simulink model "Ship_Control_Loop_H_Infinity_Standard_Controller_Comparison"  (R2024a)
settings: Solver=VariableStepAuto  StartTime=0.0  StopTime=150  RelTol=1e-3
values from neighbouring files (symbols this model uses):
  Controller = Corrector_After_Reduction    [Aposteriori_Corrector_Order_Reduction.m]    (also in Standard_H_Infinity_Controller_Tuning.m = minreal(Controller))
  Input_Matrix_Controller_Nominal = Input_Matrix_Controller_After_Reduction    [Aposteriori_Corrector_Order_Reduction.m]
  Input_Measurement_Matrix_Controller_Nominal = Input_Measurement_Matrix_Controller_After_Reduction    [Aposteriori_Corrector_Order_Reduction.m]
  Measurement_Matrix_Controller_Nominal = Measurement_Matrix_Controller_After_Reduction    [Aposteriori_Corrector_Order_Reduction.m]
  Perturbation_Step = 10*(pi/180)    (= 0.174532925199)    [Controller_Stochastic_Optimization.m]    (also in Frequency_Responses.m)
  State_Matrix_Controller_Nominal = State_Matrix_Controller_After_Reduction    [Aposteriori_Corrector_Order_Reduction.m]
  Step_Heading_Aimed = 30*(pi/180)    (= 0.523598775598)    [Controller_Stochastic_Optimization.m]    (also in Frequency_Responses.m)
libraries: cstblocks x2, RCTblocks x2
settings Model: Creator=gerar  LastModifiedBy=gerar

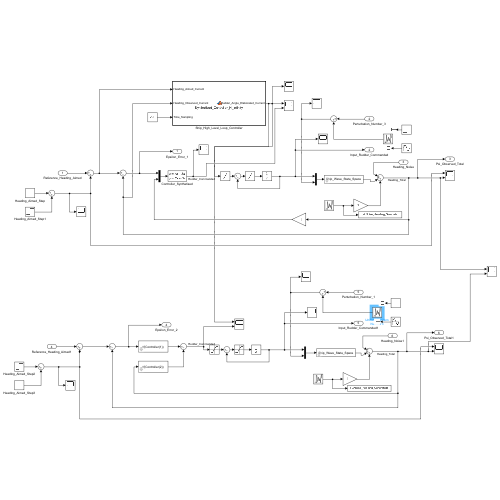
[thumbnail: Simulink's stored preview of the top-level diagram]
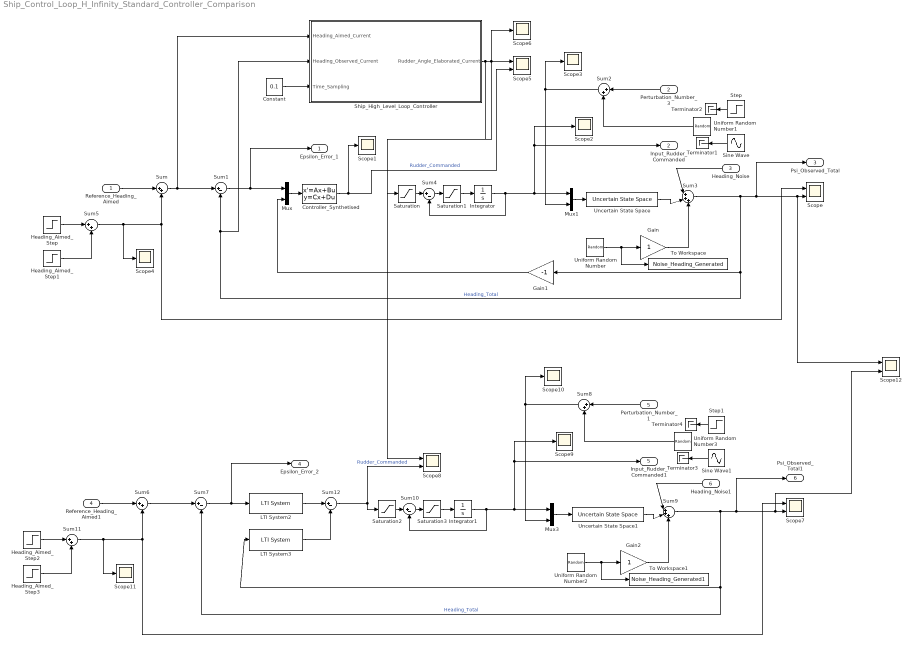
== system Ship_Control_Loop_H_Infinity_Standard_Controller_Comparison ==
  Reference_Heading_Aimed : Inport
  Perturbation_Number_3 : Inport  Port=2
  Heading_Noise : Inport  Port=3
  Reference_Heading_Aimed1 : Inport  Port=4
  Perturbation_Number_1 : Inport  Port=5
  Heading_Noise1 : Inport  Port=6
  Constant : Constant  Value=0.1
  Controller_Synthetised : StateSpace  A=State_Matrix_Controller_Nominal  B=Input_Matrix_Controller_Nominal  C=Measurement_Matrix_Controller_Nominal  D=Input_Measurement_Matrix_Controller_Nominal  InitialCondition=0
  Gain : Gain  SaturateOnIntegerOverflow=on  OutDataTypeStr=Inherit: Same as input  ParamDataTypeStr=Inherit: Same as input
  Gain1 : Gain  Gain=-1  SaturateOnIntegerOverflow=on  OutDataTypeStr=Inherit: Same as input  ParamDataTypeStr=Inherit: Same as input
  Gain2 : Gain  SaturateOnIntegerOverflow=on  OutDataTypeStr=Inherit: Same as input  ParamDataTypeStr=Inherit: Same as input
  Heading_Aimed_Step : Step  Time=0  After=Step_Heading_Aimed  SampleTime=0
  Heading_Aimed_Step1 : Step  Time=20  After=50*(pi/180)  SampleTime=0
  Heading_Aimed_Step2 : Step  Time=0  After=Step_Heading_Aimed  SampleTime=0
  Heading_Aimed_Step3 : Step  Time=20  After=50*(pi/180)  SampleTime=0
  Integrator : Integrator
  Integrator1 : Integrator
  LTI System2 : cstblocks/LTI System  sys=tf(Controller(1))  IC=[]  PadeOrder=0
  LTI System3 : cstblocks/LTI System  sys=tf(Controller(2))  IC=[]  PadeOrder=0
  Mux : Mux  Inputs=2
  Mux1 : Mux  Inputs=2
  Mux3 : Mux  Inputs=2
  Saturation : Saturate  UpperLimit=35*(pi/180)  LowerLimit=-35*(pi/180)
  Saturation1 : Saturate  UpperLimit=8*(pi/180)  LowerLimit=-8*(pi/180)
  Saturation2 : Saturate  UpperLimit=35*(pi/180)  LowerLimit=-35*(pi/180)
  Saturation3 : Saturate  UpperLimit=8*(pi/180)  LowerLimit=-8*(pi/180)
  Scope{,5,7..8,12} (5 alike) : Scope  NumInputPorts=2
  Scope{1..4,6,9..11} (8 alike) : Scope
  Ship_High_Level_Loop_Controller : MATLAB Function  TreatAsAtomicUnit=on  SystemSampleTime=0.1
  Sine Wave : Sin  Amplitude=2*(pi/180)  Frequency=0.6  SampleTime=0
  Sine Wave1 : Sin  Amplitude=2*(pi/180)  Frequency=0.6  SampleTime=0
  Step : Step  Time=10  After=Perturbation_Step  SampleTime=0
  Step1 : Step  Time=10  After=Perturbation_Step  SampleTime=0
  Sum{,2,5..6,8,11} (6 alike) : Sum  Inputs=|++
  Sum{1,4,7,10,12} (5 alike) : Sum  Inputs=|+-
  Sum3 : Sum  Inputs=|+++
  Sum9 : Sum  Inputs=|+++
  Terminator{1..4} (4 alike) : Terminator
  To Workspace : ToWorkspace  VariableName=Noise_Heading_Generated  SaveFormat=Timeseries  SampleTime=-1
  To Workspace1 : ToWorkspace  VariableName=Noise_Heading_Generated1  SaveFormat=Timeseries  SampleTime=-1
  Uncertain State Space : RCTblocks/Uncertain State Space  Tag=USS  USystem=Ship_Wave_State_Space  UValue=[]  X0=[]  uX0=[]
  Uncertain State Space1 : RCTblocks/Uncertain State Space  Tag=USS  USystem=Ship_Wave_State_Space  UValue=[]  X0=[]  uX0=[]
  Uniform Random Number : UniformRandomNumber  Minimum=-0.5*(pi/180)  Maximum=0.5*(pi/180)  SampleTime=1e-2
  Uniform Random Number1 : UniformRandomNumber  Minimum=-15*(pi/180)  Maximum=15*(pi/180)  SampleTime=1e-2
  Uniform Random Number2 : UniformRandomNumber  Minimum=-0.5*(pi/180)  Maximum=0.5*(pi/180)  SampleTime=1e-2
  Uniform Random Number3 : UniformRandomNumber  Minimum=-15*(pi/180)  Maximum=15*(pi/180)  SampleTime=1e-2
  Epsilon_Error_1 : Outport
  Input_Rudder_Commanded : Outport  Port=2
  Psi_Observed_Total : Outport  Port=3
  Epsilon_Error_2 : Outport  Port=4
  Input_Rudder_Commanded1 : Outport  Port=5
  Psi_Observed_Total1 : Outport  Port=6
  wires:
  Reference_Heading_Aimed/1 -> Sum/1
  Sum/1 -> Ship_High_Level_Loop_Controller/1(Heading_Aimed_Current), Sum1/1
  Sum1/1 -> Epsilon_Error_1/1, Mux/1
  Mux/1 -> Controller_Synthetised/1
  Controller_Synthetised/1 -> Scope5/2, Scope1/1  "Rudder_Commanded"
  Perturbation_Number_3/1 -> Sum2/1
  Sum2/1 -> Scope3/1, Mux1/2
  Mux1/1 -> Uncertain State Space/1
  Uncertain State Space/1 -> Sum3/2
  Heading_Noise/1 -> Sum3/1
  Uniform Random Number/1 -> To Workspace/1, Gain/1
  Gain/1 -> Sum3/3
  Sum3/1 -> Gain1/1, Ship_High_Level_Loop_Controller/2(Heading_Observed_Current), Sum1/2, Psi_Observed_Total/1, Scope12/1, Scope/2  "Heading_Total"
  Gain1/1 -> Mux/2
  Saturation1/1 -> Integrator/1
  Integrator/1 -> Sum4/2, Scope2/1, Input_Rudder_Commanded/1, Mux1/1
  Saturation/1 -> Sum4/1
  Sum4/1 -> Saturation1/1
  Sine Wave/1 -> Terminator1/1
  Uniform Random Number1/1 -> Sum2/2
  Step/1 -> Terminator2/1
  Heading_Aimed_Step/1 -> Sum5/1
  Heading_Aimed_Step1/1 -> Sum5/2
  Sum5/1 -> Scope4/1, Sum/2, Scope/1
  Constant/1 -> Ship_High_Level_Loop_Controller/3(Time_Sampling)
  Ship_High_Level_Loop_Controller/1(Rudder_Angle_Elaborated_Current) -> Scope8/1, Saturation/1, Scope5/1, Scope6/1
  Mux3/1 -> Uncertain State Space1/1
  Sum11/1 -> Scope11/1, Sum6/2, Scope7/1
  Uniform Random Number2/1 -> To Workspace1/1, Gain2/1
  Heading_Noise1/1 -> Sum9/1
  Uncertain State Space1/1 -> Sum9/2
  Gain2/1 -> Sum9/3
  Heading_Aimed_Step3/1 -> Sum11/2
  Saturation2/1 -> Sum10/1
  Saturation3/1 -> Integrator1/1
  Step1/1 -> Terminator4/1
  Uniform Random Number3/1 -> Sum8/2
  Sum12/1 -> Saturation2/1, Scope8/2  "Rudder_Commanded"
  Reference_Heading_Aimed1/1 -> Sum6/1
  Perturbation_Number_1/1 -> Sum8/1
  Sum7/1 -> Epsilon_Error_2/1, LTI System2/1
  Sum8/1 -> Scope10/1, Mux3/2
  Sum6/1 -> Sum7/1
  Integrator1/1 -> Sum10/2, Scope9/1, Input_Rudder_Commanded1/1, Mux3/1
  Sum10/1 -> Saturation3/1
  Sum9/1 -> LTI System3/1, Sum7/2, Psi_Observed_Total1/1, Scope12/2, Scope7/2  "Heading_Total"
  Sine Wave1/1 -> Terminator3/1
  Heading_Aimed_Step2/1 -> Sum11/1
  LTI System3/1 -> Sum12/2
  LTI System2/1 -> Sum12/1

== matlab function Ship_Control_Loop_H_Infinity_Standard_Controller_Comparison/Ship_High_Level_Loop_Controller ==
  data: Heading_Aimed_Current input; Rudder_Angle_Elaborated_Current output; Heading_Observed_Current input; Time_Sampling input
function Rudder_Angle_Elaborated_Current = Synthetized_Controller_H_Infinity(Heading_Aimed_Current,...
                                                                             Heading_Observed_Current,...
                                                                             Time_Sampling)


% This controller is based on the stochastic optimization done to find
% optimal parameters for the reduced controller of order 3 with two degrees
% of freedom.
% Heading observed persistents:
persistent Heading_Observed_Previous;
persistent Heading_Observed_Previous_Previous;
persistent Heading_Observed_Previous_Previous_Previous;
% Heading aimed persistents:
persistent Heading_Aimed_Previous;
persistent Heading_Aimed_Previous_Previous;
persistent Heading_Aimed_Previous_Previous_Previous;
% Rudder persistents:
persistent Rudder_Transfer_1_Previous;
persistent Rudder_Transfer_1_Previous_Previous;
persistent Rudder_Transfer_1_Previous_Previous_Previous;
persistent Rudder_Transfer_2_Previous;
persistent Rudder_Transfer_2_Previous_Previous;
persistent Rudder_Transfer_2_Previous_Previous_Previous;

% Persistents initialization:
if isempty(Heading_Observed_Previous)
    Heading_Observed_Previous = 0;
    Heading_Observed_Previous_Previous = 0;
    Heading_Observed_Previous_Previous_Previous = 0;
end
if isempty(Heading_Aimed_Previous)
    Heading_Aimed_Previous = 0;
    Heading_Aimed_Previous_Previous = 0;
    Heading_Aimed_Previous_Previous_Previous = 0;
end
if isempty(Rudder_Transfer_1_Previous)
    Rudder_Transfer_1_Previous = 0;
    Rudder_Transfer_1_Previous_Previous = 0;
    Rudder_Transfer_1_Previous_Previous_Previous = 0;
end
if isempty(Rudder_Transfer_2_Previous)
    Rudder_Transfer_2_Previous = 0;
    Rudder_Transfer_2_Previous_Previous = 0;
    Rudder_Transfer_2_Previous_Previous_Previous = 0;
end

% Tustin sampling:
Tustin_Sampling = 2/Time_Sampling;

% Controller coefficients:
% Numerator_Coefficient_Controller_1_1 = -1.663e-05;
% Numerator_Coefficient_Controller_1_2 = -0.4395;
% Numerator_Coefficient_Controller_1_3 = -3.978;
% Numerator_Coefficient_Controller_1_4 = -0.178;
% Denominator_Coefficient_Controller_1_1 = 1;
% Denominator_Coefficient_Controller_1_2 = 12.05;
% Denominator_Coefficient_Controller_1_3 = 14.03;
% Denominator_Coefficient_Controller_1_4 = 8.131;
% 
% Numerator_Coefficient_Controller_2_1 = -0.00014;
% Numerator_Coefficient_Controller_2_2 = -1.349;
% Numerator_Coefficient_Controller_2_3 = -17.03;
% Numerator_Coefficient_Controller_2_4 = 0.0001091;
% Denominator_Coefficient_Controller_2_1 = 1;
% Denominator_Coefficient_Controller_2_2 = 12.05;
% Denominator_Coefficient_Controller_2_3 = 14.03;
% Denominator_Coefficient_Controller_2_4 = 8.131;

Numerator_Coefficient_Controller_1_1 = 4.251e-05;
Numerator_Coefficient_Controller_1_2 = -1.03;
Numerator_Coefficient_Controller_1_3 = -1.866;
Numerator_Coefficient_Controller_1_4 = -0.1164;
Denominator_Coefficient_Controller_1_1 = 1;
Denominator_Coefficient_Controller_1_2 = 3.259;
Denominator_Coefficient_Controller_1_3 = 3.782;
Denominator_Coefficient_Controller_1_4 = 1.992;

Numerator_Coefficient_Controller_2_1 = 6.017e-05;
Numerator_Coefficient_Controller_2_2 = -2.254;
Numerator_Coefficient_Controller_2_3 = -3.937;
Numerator_Coefficient_Controller_2_4 = -6.421e-05;
Denominator_Coefficient_Controller_2_1 = 1;
Denominator_Coefficient_Controller_2_2 = 3.259;
Denominator_Coefficient_Controller_2_3 = 3.782;
Denominator_Coefficient_Controller_2_4 = 1.992;


% Coefficients calculation:
% First degree of freedom corrector:
Alpha_01 = Numerator_Coefficient_Controller_1_1*Tustin_Sampling^3 + Numerator_Coefficient_Controller_1_2*Tustin_Sampling^2 +...
           Numerator_Coefficient_Controller_1_3*Tustin_Sampling + Numerator_Coefficient_Controller_1_4;
Alpha_11 = -3*Numerator_Coefficient_Controller_1_1*Tustin_Sampling^3 - Numerator_Coefficient_Controller_1_2*Tustin_Sampling^2 +...
           Numerator_Coefficient_Controller_1_3*Tustin_Sampling + 3*Numerator_Coefficient_Controller_1_4;
Alpha_21 = 3*Numerator_Coefficient_Controller_1_1*Tustin_Sampling^3 - Numerator_Coefficient_Controller_1_2*Tustin_Sampling^2 -...
           Numerator_Coefficient_Controller_1_3*Tustin_Sampling + 3*Numerator_Coefficient_Controller_1_4;
Alpha_31 = -Numerator_Coefficient_Controller_1_1*Tustin_Sampling^3 + Numerator_Coefficient_Controller_1_2*Tustin_Sampling^2 -...
           Numerator_Coefficient_Controller_1_3*Tustin_Sampling + Numerator_Coefficient_Controller_1_4;
Beta_01 = Denominator_Coefficient_Controller_1_1*Tustin_Sampling^3 + Denominator_Coefficient_Controller_1_2*Tustin_Sampling^2 +...
          Denominator_Coefficient_Controller_1_3*Tustin_Sampling + Denominator_Coefficient_Controller_1_4;
Beta_11 = -3*Denominator_Coefficient_Controller_1_1*Tustin_Sampling^3 - Denominator_Coefficient_Controller_1_2*Tustin_Sampling^2 +...
          Denominator_Coefficient_Controller_1_3*Tustin_Sampling + 3*Denominator_Coefficient_Controller_1_4;
Beta_21 = 3*Denominator_Coefficient_Controller_1_1*Tustin_Sampling^3 - Denominator_Coefficient_Controller_1_2*Tustin_Sampling^2 -...
          Denominator_Coefficient_Controller_1_3*Tustin_Sampling + 3*Denominator_Coefficient_Controller_1_4;
Beta_31 = -Denominator_Coefficient_Controller_1_1*Tustin_Sampling^3 + Denominator_Coefficient_Controller_1_2*Tustin_Sampling^2 -...
          Denominator_Coefficient_Controller_1_3*Tustin_Sampling + Denominator_Coefficient_Controller_1_4;

% Second degree of freedom corrector:
Alpha_02 = Numerator_Coefficient_Controller_2_1*Tustin_Sampling^3 + Numerator_Coefficient_Controller_2_2*Tustin_Sampling^2 +...
           Numerator_Coefficient_Controller_2_3*Tustin_Sampling + Numerator_Coefficient_Controller_2_4;
Alpha_12 = -3*Numerator_Coefficient_Controller_2_1*Tustin_Sampling^3 - Numerator_Coefficient_Controller_2_2*Tustin_Sampling^2 +...
           Numerator_Coefficient_Controller_2_3*Tustin_Sampling + 3*Numerator_Coefficient_Controller_2_4;
Alpha_22 = 3*Numerator_Coefficient_Controller_2_1*Tustin_Sampling^3 - Numerator_Coefficient_Controller_2_2*Tustin_Sampling^2 -...
           Numerator_Coefficient_Controller_2_3*Tustin_Sampling + 3*Numerator_Coefficient_Controller_2_4;
Alpha_32 = -Numerator_Coefficient_Controller_2_1*Tustin_Sampling^3 + Numerator_Coefficient_Controller_2_2*Tustin_Sampling^2 -...
           Numerator_Coefficient_Controller_2_3*Tustin_Sampling + Numerator_Coefficient_Controller_2_4;
Beta_02 = Denominator_Coefficient_Controller_2_1*Tustin_Sampling^3 + Denominator_Coefficient_Controller_2_2*Tustin_Sampling^2 +...
          Denominator_Coefficient_Controller_2_3*Tustin_Sampling + Denominator_Coefficient_Controller_2_4;
Beta_12 = -3*Denominator_Coefficient_Controller_2_1*Tustin_Sampling^3 - Denominator_Coefficient_Controller_2_2*Tustin_Sampling^2 +...
          Denominator_Coefficient_Controller_2_3*Tustin_Sampling + 3*Denominator_Coefficient_Controller_2_4;
Beta_22 = 3*Denominator_Coefficient_Controller_2_1*Tustin_Sampling^3 - Denominator_Coefficient_Controller_2_2*Tustin_Sampling^2 -...
          Denominator_Coefficient_Controller_2_3*Tustin_Sampling + 3*Denominator_Coefficient_Controller_2_4;
Beta_32 = -Denominator_Coefficient_Controller_2_1*Tustin_Sampling^3 + Denominator_Coefficient_Controller_2_2*Tustin_Sampling^2 -...
          Denominator_Coefficient_Controller_2_3*Tustin_Sampling + Denominator_Coefficient_Controller_2_4;

% Error determination:
Error_Current = Heading_Aimed_Current - Heading_Observed_Current;
Error_Previous = Heading_Aimed_Previous - Heading_Observed_Previous;
Error_Previous_Previous = Heading_Aimed_Previous_Previous - Heading_Observed_Previous_Previous;
Error_Previous_Previous_Previous = Heading_Aimed_Previous_Previous_Previous - Heading_Observed_Previous_Previous_Previous;

% Rudder angle controller 1:
Rudder_Angle_Transfer_Error_1 = (Alpha_01/Beta_01)*Error_Current + (Alpha_11/Beta_01)*Error_Previous + (Alpha_21/Beta_01)*Error_Previous_Previous + ...
                                (Alpha_31/Beta_01)*Error_Previous_Previous_Previous - (Beta_11/Beta_01)*Rudder_Transfer_1_Previous - (Beta_21/Beta_01)*Rudder_Transfer_1_Previous_Previous -...
                                (Beta_31/Beta_01)*Rudder_Transfer_1_Previous_Previous_Previous;

% Rudder angle controller 2:
Rudder_Angle_Transfer_Heading_2 = (Alpha_02/Beta_02)*Heading_Observed_Current + (Alpha_12/Beta_02)*Heading_Observed_Previous + (Alpha_22/Beta_02)*Heading_Observed_Previous_Previous + ...
                                  (Alpha_32/Beta_02)*Heading_Observed_Previous_Previous_Previous - (Beta_12/Beta_02)*Rudder_Transfer_2_Previous - (Beta_22/Beta_02)*Rudder_Transfer_2_Previous_Previous -...
                                  (Beta_32/Beta_02)*Rudder_Transfer_2_Previous_Previous_Previous;

% Rudder angle final:
Rudder_Angle_Elaborated_Current = Rudder_Angle_Transfer_Error_1 - Rudder_Angle_Transfer_Heading_2;

% % Same denominator of the controller:
% Rudder_Angle_Elaborated_Current = (Alpha_01/Beta_01)*Error_Current + (Alpha_11/Beta_01)*Error_Previous + (Alpha_21/Beta_01)*Error_Previous_Previous + ...
%                                   (Alpha_31/Beta_01)*Error_Previous_Previous_Previous

% Persistents update:
Rudder_Transfer_1_Previous_Previous_Previous = Rudder_Transfer_1_Previous_Previous;
Rudder_Transfer_1_Previous_Previous = Rudder_Transfer_1_Previous;
Rudder_Transfer_1_Previous = Rudder_Angle_Transfer_Error_1;

Rudder_Transfer_2_Previous_Previous_Previous = Rudder_Transfer_2_Previous_Previous;
Rudder_Transfer_2_Previous_Previous = Rudder_Transfer_2_Previous;
Rudder_Transfer_2_Previous = Rudder_Angle_Transfer_Heading_2;

Heading_Aimed_Previous_Previous_Previous = Heading_Aimed_Previous_Previous;
Heading_Aimed_Previous_Previous = Heading_Aimed_Previous;
Heading_Aimed_Previous = Heading_Aimed_Current;

Heading_Observed_Previous_Previous_Previous = Heading_Observed_Previous_Previous;
Heading_Observed_Previous_Previous = Heading_Observed_Previous;
Heading_Observed_Previous = Heading_Observed_Current;

end
